simulink model "PX41s"  (R2015b)
settings: Solver=VariableStepAuto  StartTime=0.0  StopTime=20  RelTol=1e-3
settings Model: Creator=xmax1946  LastModifiedBy=xmax1946

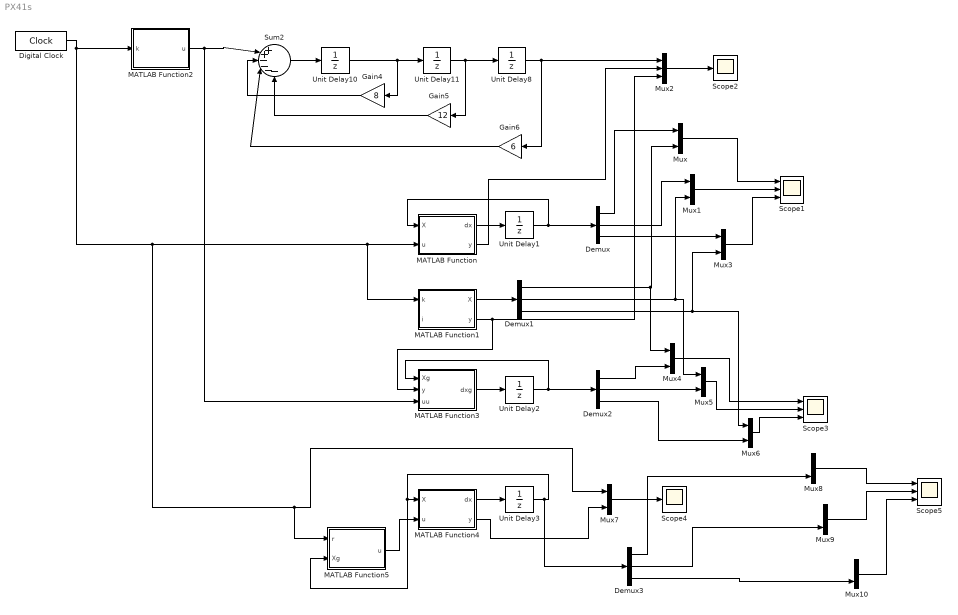
== system PX41s ==
  Demux{,1..3} (4 alike) : Demux  Outputs=3
  Digital Clock : DigitalClock
  Gain4 : Gain  Gain=8
  Gain5 : Gain  Gain=12
  Gain6 : Gain  Gain=6
  MATLAB Function : MATLAB Function  TreatAsAtomicUnit=on
  MATLAB Function1 : MATLAB Function  TreatAsAtomicUnit=on
  MATLAB Function2 : MATLAB Function  TreatAsAtomicUnit=on
  MATLAB Function3 : MATLAB Function  TreatAsAtomicUnit=on
  MATLAB Function4 : MATLAB Function  TreatAsAtomicUnit=on
  MATLAB Function5 : MATLAB Function  TreatAsAtomicUnit=on
  Mux{,1,3..10} (10 alike) : Mux  Inputs=2
  Mux2 : Mux  Inputs=3
  Scope1 : Scope  NumInputPorts=3
  Scope2 : Scope
  Scope3 : Scope  NumInputPorts=3
  Scope4 : Scope
  Scope5 : Scope  NumInputPorts=3
  Sum2 : Sum  Inputs=|++----
  Unit Delay1 : UnitDelay  InitialCondition=[-1.83333;1;0]
  Unit Delay10 : UnitDelay  InitialCondition=2
  Unit Delay11 : UnitDelay  InitialCondition=-1
  Unit Delay2 : UnitDelay  InitialCondition=[-1.9;1.1;.1]
  Unit Delay3 : UnitDelay  InitialCondition=[-1.83333;1;0]
  Unit Delay8 : UnitDelay  InitialCondition=1
  wires:
  Mux2/1 -> Scope2/1
  Unit Delay10/1 -> Unit Delay11/1, Gain4/1
  Sum2/1 -> Unit Delay10/1
  Gain4/1 -> Sum2/3
  Unit Delay11/1 -> Gain5/1, Unit Delay8/1
  Unit Delay8/1 -> Mux2/1, Gain6/1
  Gain6/1 -> Sum2/4
  Gain5/1 -> Sum2/6
  MATLAB Function/1(dx) -> Unit Delay1/1
  Unit Delay1/1 -> Demux/1, MATLAB Function/1(X)
  MATLAB Function/2(y) -> Mux2/2
  MATLAB Function1/2(y) -> MATLAB Function3/2(y), Mux2/3
  MATLAB Function2/1(u) -> MATLAB Function3/3(uu), Sum2/2
  MATLAB Function1/1(X) -> Demux1/1
  Demux/1 -> Mux/1
  Demux1/1 -> Mux4/1, Mux/2
  Demux/2 -> Mux1/1
  Demux1/2 -> Mux5/1, Mux1/2
  Demux/3 -> Mux3/1
  Demux1/3 -> Mux3/2, Mux6/1
  Mux/1 -> Scope1/1
  Mux1/1 -> Scope1/2
  Mux3/1 -> Scope1/3
  MATLAB Function3/1(dxg) -> Unit Delay2/1
  Unit Delay2/1 -> Demux2/1, MATLAB Function3/1(Xg)
  Mux4/1 -> Scope3/1
  Mux5/1 -> Scope3/2
  Mux6/1 -> Scope3/3
  Demux2/1 -> Mux4/2
  Demux2/2 -> Mux5/2
  Demux2/3 -> Mux6/2
  MATLAB Function4/1(dx) -> Unit Delay3/1
  Unit Delay3/1 -> Demux3/1, MATLAB Function5/2(Xg), MATLAB Function4/1(X)
  MATLAB Function5/1(u) -> MATLAB Function4/2(u)
  Digital Clock/1 -> MATLAB Function2/1(k), MATLAB Function5/1(r), Mux7/1, MATLAB Function1/1(k), MATLAB Function/2(u)
  Mux7/1 -> Scope4/1
  MATLAB Function4/2(y) -> Mux7/2
  Mux8/1 -> Scope5/1
  Mux9/1 -> Scope5/2
  Mux10/1 -> Scope5/3
  Demux3/1 -> Mux8/2
  Demux3/2 -> Mux9/2
  Demux3/3 -> Mux10/2

== matlab function PX41s/MATLAB Function1 ==
  data: k input; X output; y output; i input
function [X,y]=fc(k,i)
dx=[0.037037037037037037037037037037037*k + 0.00087237881159691507707423013709583*(-6.227871411936590536172105084984)^k - (- 0.886064294031704731913947457508 + 0.42225714317988059676973416764026i)^k*(0.89582418666231423257283066788062 - 0.68275413319207673651259547734736i) - (- 0.886064294031704731913947457508 - 0.42225714317988059676973416764026i)^k*(0.89582418666231423257283066788062 + 0.68275413319207673651259547734736i) - 0.042524005486968449931412894375857;
 0.037037037037037037037037037037037*k - 0.0054330630611236444032041979331453*(-6.227871411936590536172105084984)^k + (- 0.886064294031704731913947457508 + 0.42225714317988059676973416764026i)^k*(0.50546001575552752864879002763599 - 0.98323222087553487959987113894892i) + (- 0.886064294031704731913947457508 - 0.42225714317988059676973416764026i)^k*(0.50546001575552752864879002763599 + 0.98323222087553487959987113894892i) - 0.0054869684499314128943758573388203;
   0.037037037037037037037037037037037*k + 0.033836418117620645960320233756749*(-6.227871411936590536172105084984)^k - (- 0.886064294031704731913947457508 + 0.42225714317988059676973416764026i)^k*(0.032693243352363135051490706727489 - 1.0846410659038924789194810835989i) - (- 0.886064294031704731913947457508 - 0.42225714317988059676973416764026i)^k*(0.032693243352363135051490706727489 + 1.0846410659038924789194810835989i) + 0.0315500685871056241426611796982];
C=[0,1,1];
X=real(dx);
y=C*X;

== matlab function PX41s/MATLAB Function ==
  data: X input; dx output; u input; y output
function [dx,y] = fcn(X,u)
A=[0,1,0
   0,0,1
   -6,-12,-8];
B=[0;0;1];
C=[0,1,1];

dx=A*X+B*u;
y=C*X;

== matlab function PX41s/MATLAB Function2 ==
  data: u output; k input
function u = fcn(k)
uk2=k+2;
uk1=k+1;
u=uk1+uk2;

== matlab function PX41s/MATLAB Function3 ==
  data: Xg input; y input; uu input; dxg output
function dxg =fcn(Xg,y,uu)
A=[0,1,0
   0,0,1
   -6,-12,-8];
B=[0;0;1];
C=[0,1,1];
Ll=[-1;2;-10];
dxg=A*Xg+B*uu+Ll*(y-C*Xg);

== matlab function PX41s/MATLAB Function4 ==
  data: X input; dx output; u input; y output
function [dx,y] = fcn(X,u)
A=[0,1,0
   0,0,1
   -6,-12,-8];
B=[0;0;1];
C=[0,1,1];

dx=A*X+B*u;
y=C*X;

== matlab function PX41s/MATLAB Function5 ==
  data: r input; u output; Xg input
function u = fcn(r,Xg)
K=[-6,-12,-8];
u=r-K*Xg;
